simulink model "ComparisionBlock"  (R2018a)
settings: Solver=ode4  StartTime=0.0  StopTime=20  FixedStep=0.005  RelTol=1e-3
libraries: fuzblock x2
settings Model: Creator=dell  LastModifiedBy=dell

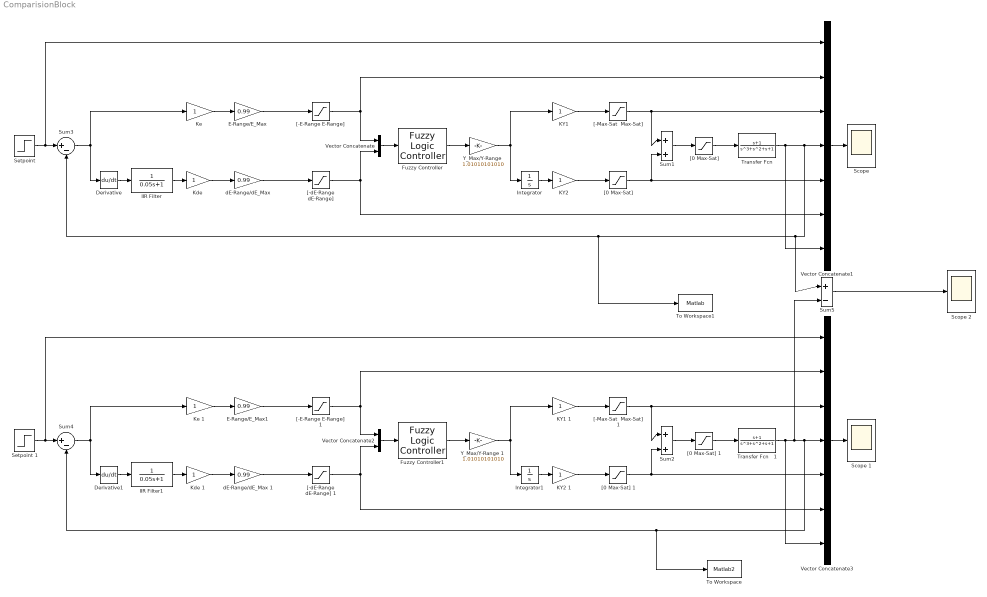
== system ComparisionBlock ==
  "    Transfer Fcn   " : TransferFcn  Numerator=[1 1]  Denominator=[1 1 1 1]
  "    Transfer Fcn   1" : TransferFcn  Numerator=[1 1]  Denominator=[1 1 1 1]
  Derivative : Derivative
  Derivative1 : Derivative
  E-Range/E_Max : Gain  Gain=0.99
  E-Range/E_Max1 : Gain  Gain=0.99
  Fuzzy Controller : fuzblock/Fuzzy Logic  Controller  FIS='1.fis'  OutputSampleNumber=1000  DataType=double  FuzzifiedInputs=off  RuleFiringStrengths=off  RuleOutputs=off  AggregatedOutputs=off  SimulateUsing=Interpreted execution  OutOfRangeInputValueMessage=none  NoRuleFiredMessage=none  EmptyOutputFuzzySetMessage=none
  Fuzzy Controller1 : fuzblock/Fuzzy Logic  Controller  FIS='1.fis'  OutputSampleNumber=10  DataType=double  FuzzifiedInputs=off  RuleFiringStrengths=off  RuleOutputs=off  AggregatedOutputs=off  SimulateUsing=Interpreted execution  OutOfRangeInputValueMessage=none  NoRuleFiredMessage=none  EmptyOutputFuzzySetMessage=none
  IIR Filter : TransferFcn  Denominator=[0.05 1]
  IIR Filter1 : TransferFcn  Denominator=[0.05 1]
  Integrator : Integrator
  Integrator1 : Integrator
  "KY1 " : Gain
  KY1 1 : Gain
  "KY2 " : Gain
  KY2 1 : Gain
  "Kde " : Gain
  Kde 1 : Gain
  "Ke " : Gain
  Ke 1 : Gain
  "Scope " : Scope
  Scope 1 : Scope
  Scope 2 : Scope
  "Setpoint " : Step  Time=0  After=50  SampleTime=0  VectorParams1D=off
  Setpoint 1 : Step  Time=0  After=50  SampleTime=0  VectorParams1D=off
  Sum1 : Sum  Inputs=|++
  Sum2 : Sum  Inputs=|++
  Sum3 : Sum  Inputs=|+-
  Sum4 : Sum  Inputs=|+-
  Sum5 : Sum  Inputs=|+-
  To Workspace : ToWorkspace  VariableName=Matlab2  SaveFormat=Timeseries  SampleTime=-1
  To Workspace1 : ToWorkspace  VariableName=Matlab  SaveFormat=Timeseries  SampleTime=-1
  Vector Concatenate : Concatenate
  Vector Concatenate1 : Concatenate  NumInputs=7
  Vector Concatenate2 : Concatenate
  Vector Concatenate3 : Concatenate  NumInputs=7
  "Y_Max/Y-Range " : Gain  Gain=1.01010101010
  Y_Max/Y-Range 1 : Gain  Gain=1.01010101010
  "[-E-Range E-Range] " : Saturate  UpperLimit=99  LowerLimit=-99  LinearizeAsGain=off  OutMin=[-100]  OutMax=[100]
  "[-E-Range E-Range] 1" : Saturate  UpperLimit=99  LowerLimit=-99  LinearizeAsGain=off  OutMin=[-100]  OutMax=[100]
  "[-Max-Sat  Max-Sat] " : Saturate  UpperLimit=100  LowerLimit=-100  LinearizeAsGain=off
  "[-Max-Sat  Max-Sat] 1" : Saturate  UpperLimit=100  LowerLimit=-100  LinearizeAsGain=off
  "[-dE-Range dE-Range] " : Saturate  UpperLimit=99  LowerLimit=-99  LinearizeAsGain=off
  "[-dE-Range dE-Range] 1" : Saturate  UpperLimit=99  LowerLimit=-99  LinearizeAsGain=off
  [0 Max-Sat] {,,1,1} (4 alike) : Saturate  UpperLimit=100  LowerLimit=0  LinearizeAsGain=off
  "dE-Range/dE_Max " : Gain  Gain=0.99
  dE-Range/dE_Max 1 : Gain  Gain=0.99
  wires:
  "Setpoint "/1 -> Vector Concatenate1/1, Sum3/1
  E-Range/E_Max/1 -> "[-E-Range E-Range] "/1
  IIR Filter/1 -> "Kde "/1
  "[-E-Range E-Range] "/1 -> Vector Concatenate1/2, Vector Concatenate/1
  Integrator/1 -> "KY2 "/1
  Fuzzy Controller/1 -> "Y_Max/Y-Range "/1
  "[0 Max-Sat] "/1 -> Vector Concatenate1/5, Sum1/2
  "[-dE-Range dE-Range] "/1 -> Vector Concatenate1/6, Vector Concatenate/2
  "Y_Max/Y-Range "/1 -> "KY1 "/1, Integrator/1
  Derivative/1 -> IIR Filter/1
  "KY2 "/1 -> "[0 Max-Sat] "/1
  Vector Concatenate/1 -> Fuzzy Controller/1
  "Kde "/1 -> "dE-Range/dE_Max "/1
  "[-Max-Sat  Max-Sat] "/1 -> Vector Concatenate1/3, Sum1/1
  "KY1 "/1 -> "[-Max-Sat  Max-Sat] "/1
  "[0 Max-Sat] "/1 -> "    Transfer Fcn   "/1
  "    Transfer Fcn   "/1 -> Vector Concatenate1/7, Vector Concatenate1/4, To Workspace1/1, Sum3/2, Sum5/1
  "dE-Range/dE_Max "/1 -> "[-dE-Range dE-Range] "/1
  Sum1/1 -> "[0 Max-Sat] "/1
  "Ke "/1 -> E-Range/E_Max/1
  Sum3/1 -> Derivative/1, "Ke "/1
  Vector Concatenate1/1 -> "Scope "/1
  Kde 1/1 -> dE-Range/dE_Max 1/1
  Vector Concatenate2/1 -> Fuzzy Controller1/1
  Derivative1/1 -> IIR Filter1/1
  KY2 1/1 -> "[0 Max-Sat] 1"/1
  Integrator1/1 -> KY2 1/1
  "[-E-Range E-Range] 1"/1 -> Vector Concatenate3/2, Vector Concatenate2/1
  "[0 Max-Sat] 1"/1 -> Vector Concatenate3/5, Sum2/2
  Setpoint 1/1 -> Vector Concatenate3/1, Sum4/1
  IIR Filter1/1 -> Kde 1/1
  E-Range/E_Max1/1 -> "[-E-Range E-Range] 1"/1
  Vector Concatenate3/1 -> Scope 1/1
  Sum4/1 -> Derivative1/1, Ke 1/1
  dE-Range/dE_Max 1/1 -> "[-dE-Range dE-Range] 1"/1
  Ke 1/1 -> E-Range/E_Max1/1
  Sum2/1 -> "[0 Max-Sat] 1"/1
  "    Transfer Fcn   1"/1 -> Vector Concatenate3/7, Sum5/2, Vector Concatenate3/4, To Workspace/1, Sum4/2
  "[0 Max-Sat] 1"/1 -> "    Transfer Fcn   1"/1
  KY1 1/1 -> "[-Max-Sat  Max-Sat] 1"/1
  Fuzzy Controller1/1 -> Y_Max/Y-Range 1/1
  "[-Max-Sat  Max-Sat] 1"/1 -> Vector Concatenate3/3, Sum2/1
  "[-dE-Range dE-Range] 1"/1 -> Vector Concatenate3/6, Vector Concatenate2/2
  Y_Max/Y-Range 1/1 -> KY1 1/1, Integrator1/1
  Sum5/1 -> Scope 2/1
